simulink model "observer_design"  (R2018a)
settings: Solver=VariableStepAuto  StartTime=0.0  StopTime=20  RelTol=1e-3
model workspace (MATLAB code in the model file):
  | Cr=198000;
  | Cf=470000;
  | cf=Cf;
  | cr=Cr;
  | Mz=1000;
  | lf=3.67;
  | lr=1.93;
  | m=9950;
  | J=5;
  | Iz=5;
  | v=50;
  | nu=1;
  | mu=nu;
  | a0=(Cf*Cr*(lf+lr)^2)+(Cr*lr-Cf*lf)*m*v^2;
  | a1=(Cf*(J+lf^2*m)+Cr*(J+lr^2*m))*v;
  | a2=J*m*v^2;
  | b0=(Cf*Cr*(lf+lr))*v;
  | b1=(Cf*lf)*m*v^2;
  | 
  | A1=[(-mu*cf-mu*cr)/(m*v) -1+((mu*cr*lr-mu*cf*lf)/(m*v^2))];
  | A2=[(mu*cr*lr-mu*cf*lf)/(Iz) (-mu*cf*lf^2-mu*cr*lr^2)/(Iz*v)];
  | A=[A1;A2];
  | B=[(mu*cf)/(m*v);(mu*cf*lf)/(Iz)];
  | C=[0 1];
  | D=[0];
  | e=[-5+8.6i,-5-8.6i];
  | k=place(A,B,e);
  | p=[-5+8.6i,-5-8.6i];
  | L=acker(A',C',p)';
  | L=L;
  | x0=[0,0];
  | Ahat = A;
  | Bhat = [B, L];
  | Chat=[1 0;0 1];
  | Dhat = [0, 0; 0, 0];
  | xhat0 = [5, 5];
values from neighbouring files (symbols this model uses):
  DeltaF = 1    [LQR.m]
settings Model: Creator=uzeyi  LastModifiedBy=uzeyi

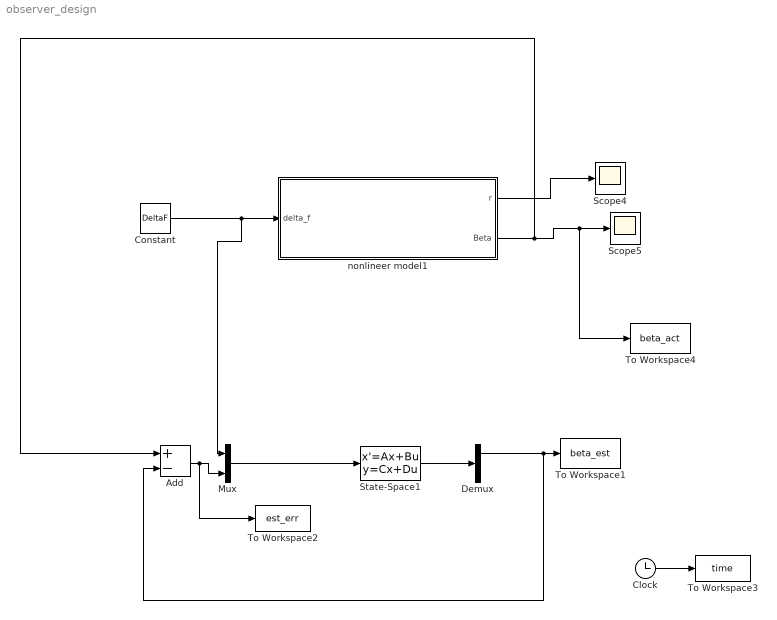
== system observer_design ==
  Add : Sum  Inputs=+-
  Clock : Clock
  Constant : Constant  Value=DeltaF
  Demux : Demux  Outputs=2
  Mux : Mux  Inputs=2
  Scope4 : Scope
  Scope5 : Scope
  State-Space1 : StateSpace  A=A  B=Bhat  C=Chat  D=[0 0;0 0]  InitialCondition=x0
  To Workspace1 : ToWorkspace  VariableName=beta_est  SampleTime=-1
  To Workspace2 : ToWorkspace  VariableName=est_err  SampleTime=-1
  To Workspace3 : ToWorkspace  VariableName=time  SampleTime=-1
  To Workspace4 : ToWorkspace  VariableName=beta_act  SampleTime=-1
  nonlineer model1 : Subsystem
  wires:
  Add/1 -> To Workspace2/1, Mux/2
  State-Space1/1 -> Demux/1
  Clock/1 -> To Workspace3/1
  nonlineer model1/1(r) -> Scope4/1
  nonlineer model1/2(Beta) -> Add/1, To Workspace4/1, Scope5/1
  Demux/1 -> Add/2, To Workspace1/1
  Constant/1 -> Mux/1, nonlineer model1/1(delta_f)
  Mux/1 -> State-Space1/1

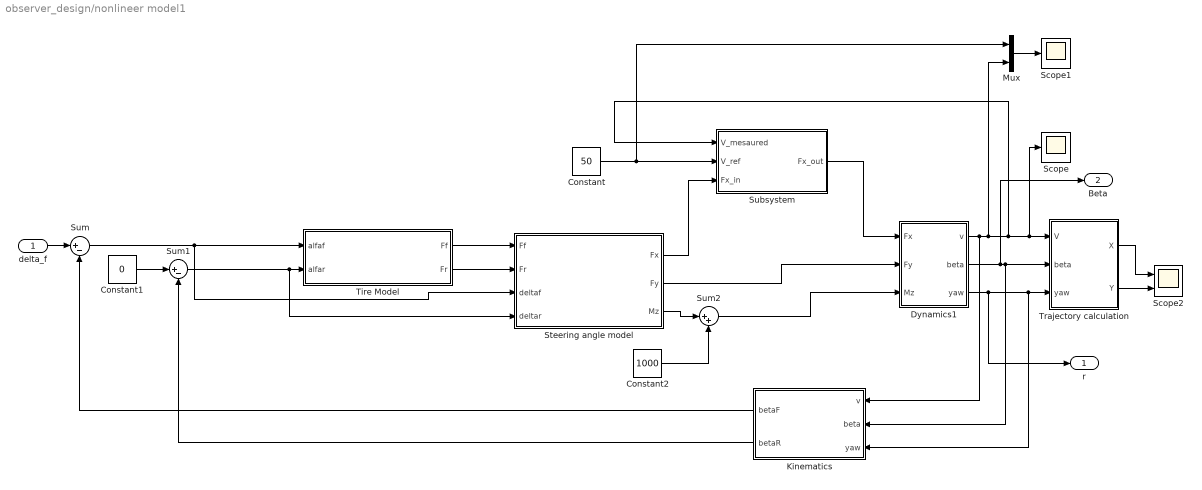
== system observer_design/nonlineer model1 ==
  delta_f : Inport
  Constant : Constant  Value=50
  Constant1 : Constant  Value=0
  Constant2 : Constant  Value=1000
  Dynamics1 : Subsystem
  "Kinematics\t\t" : Subsystem
  Mux : Mux  Inputs=2
  Scope : Scope
  Scope1 : Scope
  Scope2 : Scope  NumInputPorts=2
  Steering angle model : Subsystem
  Subsystem : Subsystem
  Sum : Sum  Inputs=|+-
  Sum1 : Sum  Inputs=|+-
  Sum2 : Sum  Inputs=|++
  Tire Model : Subsystem
  Trajectory calculation : Subsystem
  r : Outport
  Beta : Outport  Port=2
  wires:
  Tire Model/2(Fr) -> Steering angle model/2("Fr ")
  Tire Model/1(Ff) -> Steering angle model/1(Ff)
  "Kinematics\t\t"/1(betaF) -> Sum/2
  Sum/1 -> Tire Model/1(alfaf), Steering angle model/3("deltaf ")
  delta_f/1 -> Sum/1
  "Kinematics\t\t"/2(betaR) -> Sum1/2
  Constant1/1 -> Sum1/1
  Sum1/1 -> Steering angle model/4(deltar), Tire Model/2(alfar)
  Steering angle model/3(Mz) -> Sum2/1
  Constant2/1 -> Sum2/2
  Constant/1 -> Mux/1, Subsystem/2(V_ref)
  Steering angle model/1(Fx) -> Subsystem/3(Fx_in)
  Subsystem/1(Fx_out) -> Dynamics1/1(Fx)
  Steering angle model/2(Fy) -> Dynamics1/2(Fy)
  Sum2/1 -> Dynamics1/3(Mz)
  Dynamics1/3(yaw) -> r/1, "Kinematics\t\t"/3(yaw), Trajectory calculation/3(yaw)
  Dynamics1/2(beta) -> Beta/1, "Kinematics\t\t"/2(beta), Trajectory calculation/2(beta)
  Dynamics1/1(v) -> Mux/2, Subsystem/1("V_mesaured "), Scope/1, Trajectory calculation/1(V), "Kinematics\t\t"/1(v)
  Mux/1 -> Scope1/1
  Trajectory calculation/2(Y) -> Scope2/2
  Trajectory calculation/1(X) -> Scope2/1

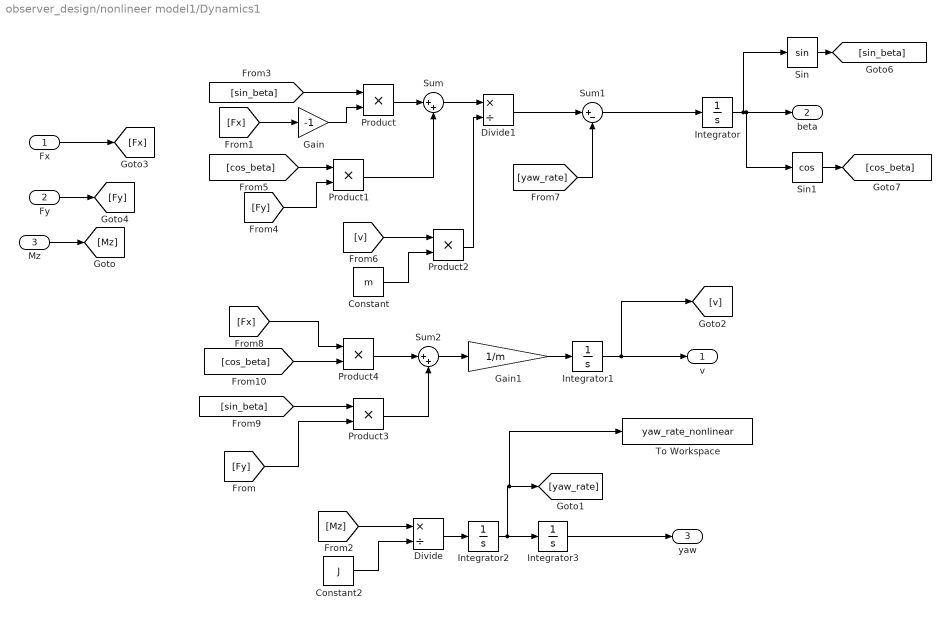
== system observer_design/nonlineer model1/Dynamics1 ==
  Fx : Inport
  Fy : Inport  Port=2
  Mz : Inport  Port=3
  Constant : Constant  Value=m
  Constant2 : Constant  Value=J
  Divide : Product  Inputs=*/
  Divide1 : Product  Inputs=*/
  Gain : Gain  Gain=-1
  Gain1 : Gain  Gain=1/m
  Integrator : Integrator
  Integrator1 : Integrator  InitialCondition=1
  Integrator2 : Integrator
  Integrator3 : Integrator
  Product{,1..4} (5 alike) : Product
  Sin : Trigonometry
  Sin1 : Trigonometry  Operator=cos
  Sum : Sum  Inputs=|++
  Sum1 : Sum  Inputs=|+-
  Sum2 : Sum  Inputs=|++
  To Workspace : ToWorkspace  VariableName=yaw_rate_nonlinear  SampleTime=-1
  v : Outport
  beta : Outport  Port=2
  yaw : Outport  Port=3
  wires:
  Fx/1 -> [Fx]
  Fy/1 -> [Fy]
  Integrator1/1 -> [v], v/1
  Integrator3/1 -> yaw/1
  Mz/1 -> [Mz]
  [Mz] -> Divide/1
  Constant2/1 -> Divide/2
  Divide/1 -> Integrator2/1
  Integrator2/1 -> To Workspace/1, [yaw_rate], Integrator3/1
  Integrator/1 -> Sin/1, beta/1, Sin1/1
  Sin/1 -> [sin_beta]
  Sin1/1 -> [cos_beta]
  [Fx] -> Gain/1
  [sin_beta] -> Product/1
  Gain/1 -> Product/2
  [cos_beta] -> Product1/1
  [Fy] -> Product1/2
  Product/1 -> Sum/1
  Product1/1 -> Sum/2
  [v] -> Product2/1
  Constant/1 -> Product2/2
  Sum/1 -> Divide1/1
  Product2/1 -> Divide1/2
  [yaw_rate] -> Sum1/2
  Divide1/1 -> Sum1/1
  Sum1/1 -> Integrator/1
  [sin_beta] -> Product3/1
  [Fy] -> Product3/2
  [cos_beta] -> Product4/2
  [Fx] -> Product4/1
  Product4/1 -> Sum2/1
  Product3/1 -> Sum2/2
  Sum2/1 -> Gain1/1
  Gain1/1 -> Integrator1/1

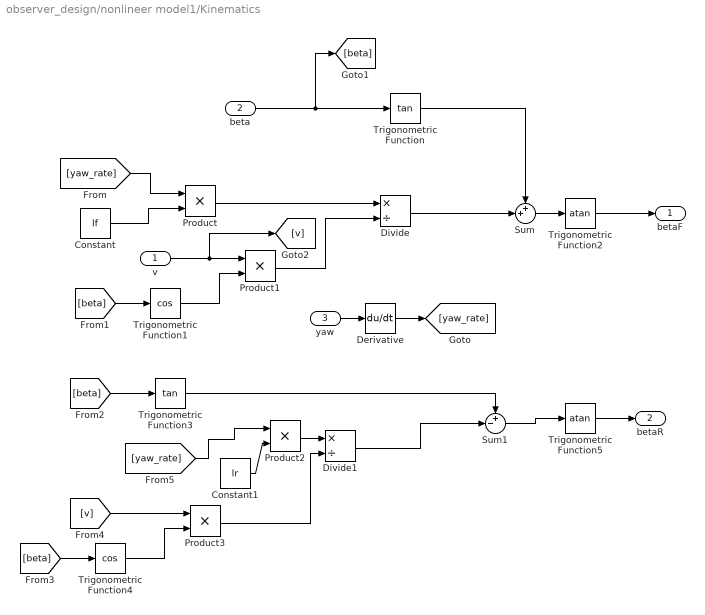
== system observer_design/nonlineer model1/Kinematics		 ==
  v : Inport
  beta : Inport  Port=2
  yaw : Inport  Port=3
  Constant : Constant  Value=lf
  Constant1 : Constant  Value=lr
  Derivative : Derivative
  Divide : Product  Inputs=*/
  Divide1 : Product  Inputs=*/
  Product{,1..3} (4 alike) : Product
  Sum : Sum  Inputs=++|
  Sum1 : Sum  Inputs=+-|
  Trigonometric Function : Trigonometry  Operator=tan
  Trigonometric Function1 : Trigonometry  Operator=cos
  Trigonometric Function2 : Trigonometry  Operator=atan
  Trigonometric Function3 : Trigonometry  Operator=tan
  Trigonometric Function4 : Trigonometry  Operator=cos
  Trigonometric Function5 : Trigonometry  Operator=atan
  betaF : Outport
  betaR : Outport  Port=2
  wires:
  beta/1 -> [beta], Trigonometric Function/1
  yaw/1 -> Derivative/1
  [yaw_rate] -> Product/1
  Constant/1 -> Product/2
  Product/1 -> Divide/1
  v/1 -> [v], Product1/1
  [beta] -> Trigonometric Function1/1
  Product1/1 -> Divide/2
  Trigonometric Function1/1 -> Product1/2
  Divide/1 -> Sum/2
  Trigonometric Function/1 -> Sum/1
  Sum/1 -> Trigonometric Function2/1
  Trigonometric Function2/1 -> betaF/1
  Derivative/1 -> [yaw_rate]
  [beta] -> Trigonometric Function3/1
  Trigonometric Function3/1 -> Sum1/1
  Divide1/1 -> Sum1/2
  [beta] -> Trigonometric Function4/1
  Trigonometric Function4/1 -> Product3/2
  Product3/1 -> Divide1/2
  [v] -> Product3/1
  Constant1/1 -> Product2/2
  [yaw_rate] -> Product2/1
  Product2/1 -> Divide1/1
  Sum1/1 -> Trigonometric Function5/1
  Trigonometric Function5/1 -> betaR/1

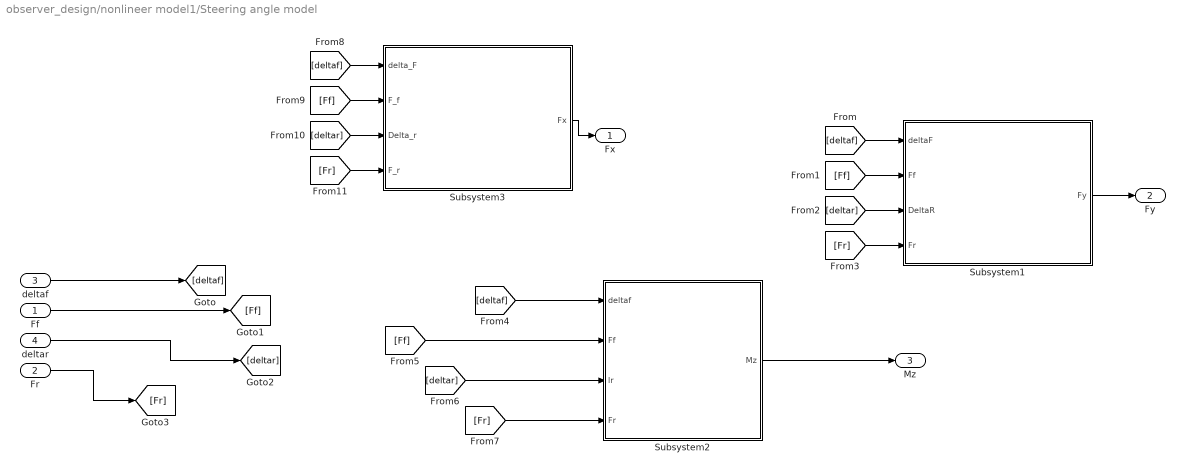
== system observer_design/nonlineer model1/Steering angle model ==
  Ff : Inport
  "Fr " : Inport  Port=2
  "deltaf " : Inport  Port=3
  deltar : Inport  Port=4
  Subsystem1 : Subsystem
  Subsystem2 : Subsystem
  Subsystem3 : Subsystem
  Fx : Outport
  Fy : Outport  Port=2
  Mz : Outport  Port=3
  wires:
  "deltaf "/1 -> [deltaf]
  Ff/1 -> [Ff]
  "Fr "/1 -> [Fr]
  deltar/1 -> [deltar]
  [deltaf] -> Subsystem1/1("deltaF ")
  [Ff] -> Subsystem1/2(Ff)
  [deltar] -> Subsystem1/3(DeltaR)
  [Fr] -> Subsystem1/4(Fr)
  Subsystem1/1(Fy) -> Fy/1
  [deltaf] -> Subsystem2/1(deltaf)
  [Ff] -> Subsystem2/2(Ff)
  [deltar] -> Subsystem2/3(lr)
  [Fr] -> Subsystem2/4(Fr)
  Subsystem2/1(Mz) -> Mz/1
  [deltaf] -> Subsystem3/1(delta_F)
  [Ff] -> Subsystem3/2(F_f)
  [deltar] -> Subsystem3/3(Delta_r)
  [Fr] -> Subsystem3/4(F_r)
  Subsystem3/1(Fx) -> Fx/1

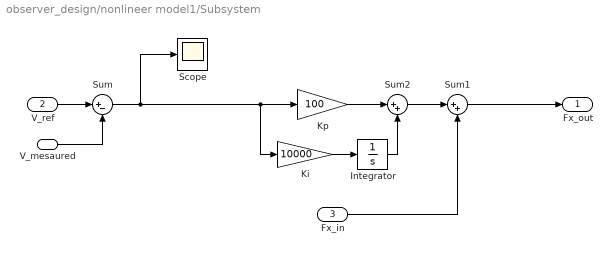
== system observer_design/nonlineer model1/Subsystem ==
  "V_mesaured " : Inport
  V_ref : Inport  Port=2
  Fx_in : Inport  Port=3
  Integrator : Integrator
  Ki : Gain  Gain=10000
  Kp : Gain  Gain=100
  Scope : Scope
  Sum : Sum  Inputs=|+-
  Sum1 : Sum  Inputs=|++
  Sum2 : Sum  Inputs=|++
  Fx_out : Outport
  wires:
  V_ref/1 -> Sum/1
  "V_mesaured "/1 -> Sum/2
  Sum/1 -> Ki/1, Kp/1, Scope/1
  Sum1/1 -> Fx_out/1
  Fx_in/1 -> Sum1/2
  Ki/1 -> Integrator/1
  Kp/1 -> Sum2/1
  Sum2/1 -> Sum1/1
  Integrator/1 -> Sum2/2

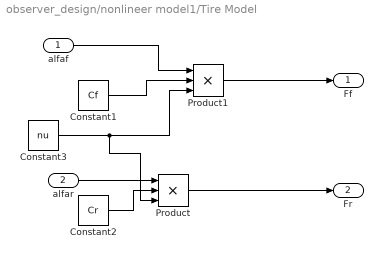
== system observer_design/nonlineer model1/Tire Model ==
  alfaf : Inport
  alfar : Inport  Port=2
  Constant1 : Constant  Value=Cf
  Constant2 : Constant  Value=Cr
  Constant3 : Constant  Value=nu
  Product : Product  Inputs=3
  Product1 : Product  Inputs=3
  Ff : Outport
  Fr : Outport  Port=2
  wires:
  alfar/1 -> Product/1
  Constant2/1 -> Product/2
  Constant1/1 -> Product1/2
  alfaf/1 -> Product1/1
  Product1/1 -> Ff/1
  Product/1 -> Fr/1
  Constant3/1 -> Product/3, Product1/3

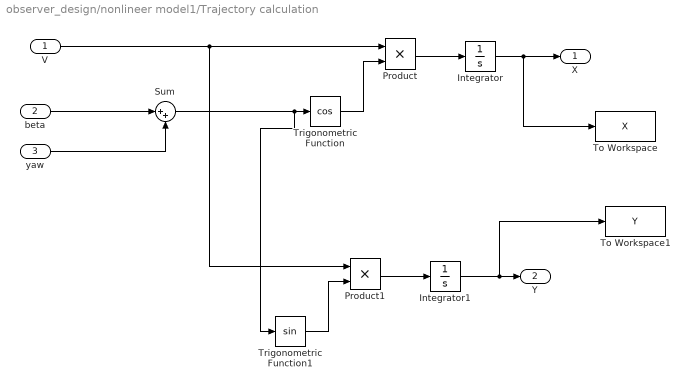
== system observer_design/nonlineer model1/Trajectory calculation ==
  V : Inport
  beta : Inport  Port=2
  yaw : Inport  Port=3
  Integrator : Integrator
  Integrator1 : Integrator
  Product : Product
  Product1 : Product
  Sum : Sum  Inputs=|++
  To Workspace : ToWorkspace  VariableName=X  SampleTime=-1
  To Workspace1 : ToWorkspace  VariableName=Y  SampleTime=-1
  Trigonometric Function : Trigonometry  Operator=cos
  Trigonometric Function1 : Trigonometry
  X : Outport
  Y : Outport  Port=2
  wires:
  V/1 -> Product1/1, Product/1
  beta/1 -> Sum/1
  Sum/1 -> Trigonometric Function1/1, Trigonometric Function/1
  Trigonometric Function/1 -> Product/2
  Product/1 -> Integrator/1
  Trigonometric Function1/1 -> Product1/2
  Product1/1 -> Integrator1/1
  Integrator1/1 -> To Workspace1/1, Y/1
  Integrator/1 -> To Workspace/1, X/1
  yaw/1 -> Sum/2

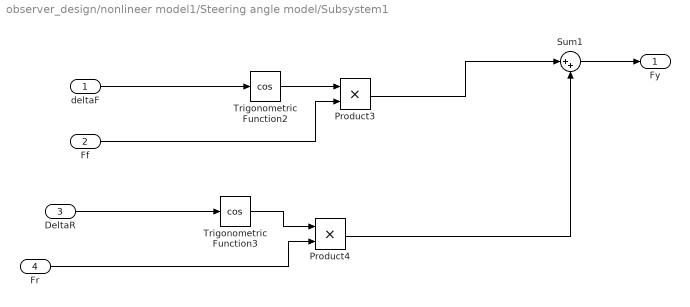
== system observer_design/nonlineer model1/Steering angle model/Subsystem1 ==
  "deltaF " : Inport
  Ff : Inport  Port=2
  DeltaR : Inport  Port=3
  Fr : Inport  Port=4
  Product3 : Product
  Product4 : Product
  Sum1 : Sum  Inputs=|++
  Trigonometric Function2 : Trigonometry  Operator=cos
  Trigonometric Function3 : Trigonometry  Operator=cos
  Fy : Outport
  wires:
  Product3/1 -> Sum1/1
  Product4/1 -> Sum1/2
  DeltaR/1 -> Trigonometric Function3/1
  Sum1/1 -> Fy/1
  Trigonometric Function2/1 -> Product3/1
  Trigonometric Function3/1 -> Product4/1
  Fr/1 -> Product4/2
  "deltaF "/1 -> Trigonometric Function2/1
  Ff/1 -> Product3/2

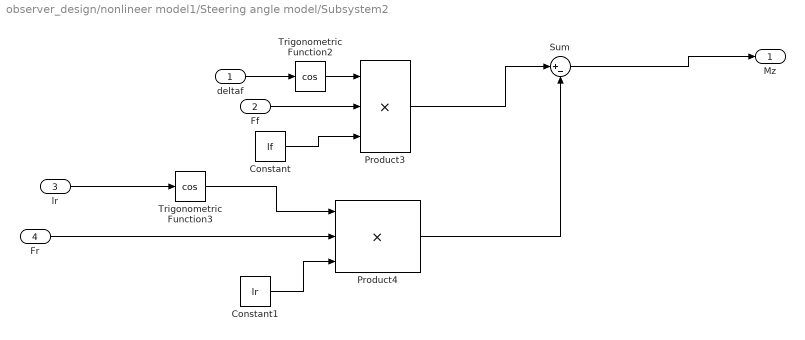
== system observer_design/nonlineer model1/Steering angle model/Subsystem2 ==
  deltaf : Inport
  Ff : Inport  Port=2
  lr : Inport  Port=3
  Fr : Inport  Port=4
  Constant : Constant  Value=lf
  Constant1 : Constant  Value=lr
  Product3 : Product  Inputs=3
  Product4 : Product  Inputs=3
  Sum : Sum  Inputs=|+-
  Trigonometric Function2 : Trigonometry  Operator=cos
  Trigonometric Function3 : Trigonometry  Operator=cos
  Mz : Outport
  wires:
  Constant1/1 -> Product4/3
  Constant/1 -> Product3/3
  lr/1 -> Trigonometric Function3/1
  Product3/1 -> Sum/1
  Product4/1 -> Sum/2
  Ff/1 -> Product3/2
  Fr/1 -> Product4/2
  deltaf/1 -> Trigonometric Function2/1
  Trigonometric Function2/1 -> Product3/1
  Trigonometric Function3/1 -> Product4/1
  Sum/1 -> Mz/1

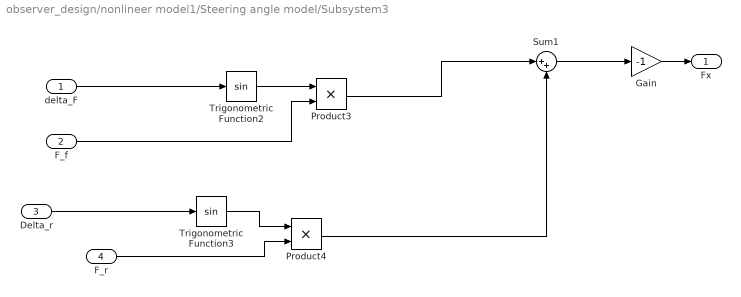
== system observer_design/nonlineer model1/Steering angle model/Subsystem3 ==
  delta_F : Inport
  F_f : Inport  Port=2
  Delta_r : Inport  Port=3
  F_r : Inport  Port=4
  Gain : Gain  Gain=-1
  Product3 : Product
  Product4 : Product
  Sum1 : Sum  Inputs=|++
  Trigonometric Function2 : Trigonometry
  Trigonometric Function3 : Trigonometry
  Fx : Outport
  wires:
  Product3/1 -> Sum1/1
  Product4/1 -> Sum1/2
  Delta_r/1 -> Trigonometric Function3/1
  Trigonometric Function2/1 -> Product3/1
  Trigonometric Function3/1 -> Product4/1
  F_r/1 -> Product4/2
  delta_F/1 -> Trigonometric Function2/1
  F_f/1 -> Product3/2
  Sum1/1 -> Gain/1
  Gain/1 -> Fx/1
